simulink model "closelooprw"  (R2024a)
settings: Solver=VariableStepAuto  StartTime=0.0  StopTime=10.0  RelTol=1e-3
undefined symbols (not defined in the file or in its folder): Error_quaternio, feedback, init, motor, sat, setPoint, x
libraries: simulink x9, aerolibconvert2 x2, sharedtransform x2
settings Model: Creator=b_ant  LastModifiedBy=b_ant

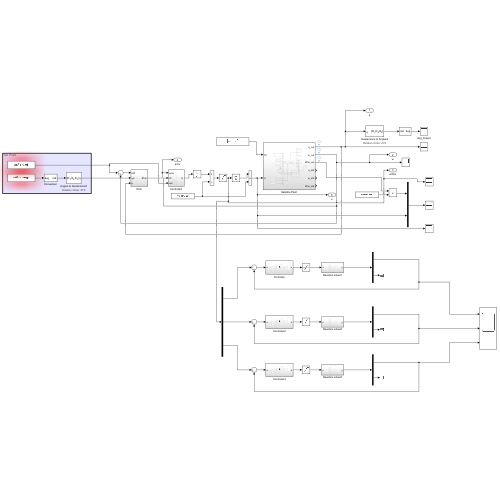
[thumbnail: Simulink's stored preview of the top-level diagram]
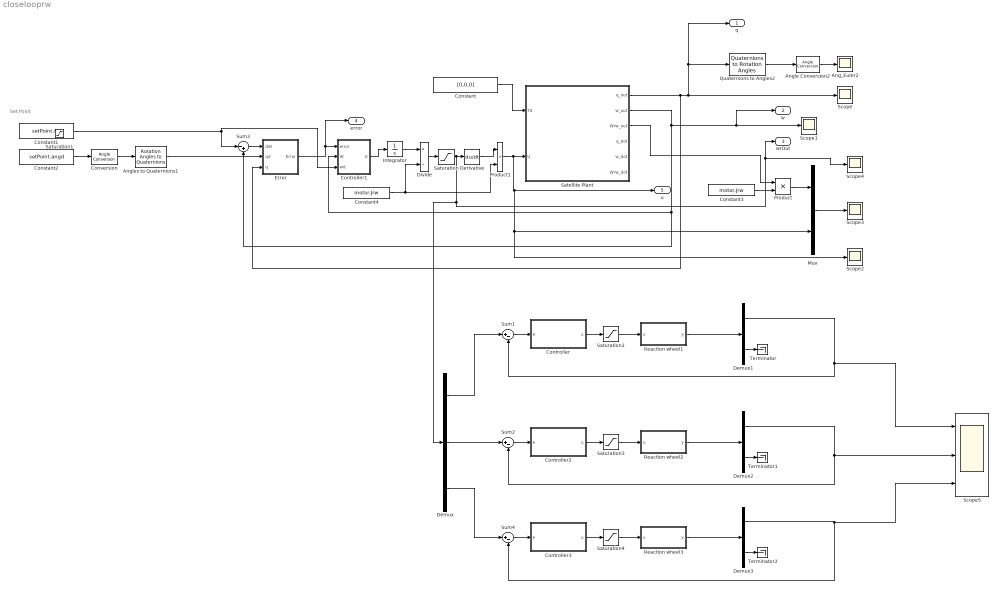
== system closelooprw ==
  note: Set Point
  Ang_Euler2 : Scope
  Angle Conversion2 : aerolibconvert2/Angle Conversion  IU=rad  OU=deg
  Angles to Quaternions1 : sharedtransform/Rotation Angles to Quaternions  rotationOrder=ZYX  aMode=aMode
  Constant : Constant  Value=[0,0,0]
  Constant1 : Constant  Value=setPoint.wd
  Constant2 : Constant  Value=setPoint.angd
  Constant3 : Constant  Value=motor.Jrw
  Constant4 : Constant  Value=motor.Jrw
  Controller : Subsystem
  Controller1 : Subsystem
  Controller2 : Subsystem
  Controller3 : Subsystem
  Conversion : aerolibconvert2/Angle Conversion  IU=deg  OU=rad
  Demux : Demux  Outputs=3
  Demux1 : Demux  Outputs=2
  Demux2 : Demux  Outputs=2
  Demux3 : Demux  Outputs=2
  Derivative : Derivative
  Divide : Product  Inputs=*/
  Error : Subsystem
  Integrator : Integrator
  Mux : Mux  Inputs=2
  Product : Product
  Product1 : Product
  Quaternions to Angles2 : sharedtransform/Quaternions to Rotation Angles  rotationOrder=ZYX  aMode=aMode
  Reaction wheel1 : Subsystem
  Reaction wheel2 : Subsystem
  Reaction wheel3 : Subsystem
  Satellite Plant : Subsystem
  Saturation : Saturate  UpperLimit=457.6253298729  LowerLimit=-457.6253298729
  Saturation{1..4} (4 alike) : Saturate  UpperLimit=12  LowerLimit=-12
  Scope{,1..4} (5 alike) : Scope
  Scope5 : Scope  NumInputPorts=3
  Sum1 : Sum  Inputs=|+-
  Sum2 : Sum  Inputs=|+-
  Sum3 : Sum  Inputs=|-+
  Sum4 : Sum  Inputs=|+-
  Terminator : Terminator
  Terminator1 : Terminator
  Terminator2 : Terminator
  q : Outport
  w : Outport  Port=2
  wrOut : Outport  Port=3
  error : Outport  Port=4
  u : Outport  Port=5
  wires:
  Reaction wheel1/1(y) -> Demux1/1
  Demux1/1 -> Scope5/1, Sum1/2
  Saturation/1 -> Demux/1, Scope4/1, wrOut/1, Derivative/1
  Sum1/1 -> Controller/1(e)
  Demux1/2 -> Terminator/1
  Derivative/1 -> Product1/1
  Product1/1 -> Scope2/1, Mux/2, u/1, Satellite Plant/2(U)
  Conversion/1 -> Angles to Quaternions1/1
  Constant/1 -> Satellite Plant/1(Td)
  Integrator/1 -> Divide/1
  Constant2/1 -> Conversion/1
  Quaternions to Angles2/1 -> Angle Conversion2/1
  Product/1 -> Mux/1
  Satellite Plant/2(w_out) -> Sum3/2, Controller1/2(W), w/1, Scope1/1
  Divide/1 -> Saturation/1
  Constant4/1 -> Product1/2, Divide/2
  Constant1/1 -> Sum3/1, Controller1/3(wd)
  Error/1(Error) -> Controller1/1(error), error/1
  Satellite Plant/3(Wrw_out) -> Product/1
  Constant3/1 -> Product/2
  Sum3/1 -> Error/1(dW)
  Controller1/1(U) -> Integrator/1
  Satellite Plant/1(q_out) -> Error/3(q), q/1, Quaternions to Angles2/1, Scope/1
  Angle Conversion2/1 -> Ang_Euler2/1
  Angles to Quaternions1/1 -> Error/2(qd)
  Mux/1 -> Scope3/1
  Controller/1(u) -> Saturation2/1
  Saturation2/1 -> Reaction wheel1/1(u)
  Controller2/1(u) -> Saturation3/1
  Saturation3/1 -> Reaction wheel2/1(u)
  Demux2/1 -> Sum2/2, Scope5/2
  Sum2/1 -> Controller2/1(e)
  Reaction wheel2/1(y) -> Demux2/1
  Controller3/1(u) -> Saturation4/1
  Saturation4/1 -> Reaction wheel3/1(u)
  Demux3/1 -> Scope5/3, Sum4/2
  Sum4/1 -> Controller3/1(e)
  Reaction wheel3/1(y) -> Demux3/1
  Demux2/2 -> Terminator1/1
  Demux3/2 -> Terminator2/1
  Demux/2 -> Sum2/1
  Demux/1 -> Sum1/1
  Demux/3 -> Sum4/1

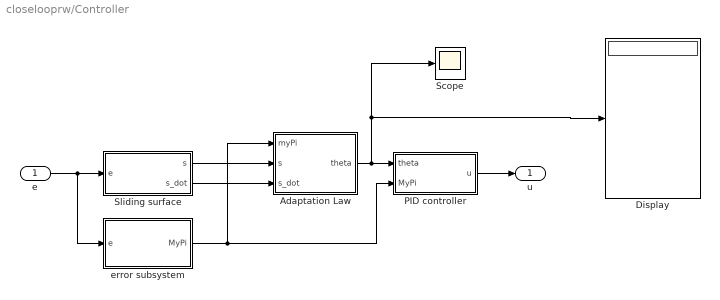
== system closelooprw/Controller ==
  e : Inport
  Adaptation Law : Subsystem  mask{alpha=x.alpha, beta=x.beta, epsilon=x.epsilon, n=x.n, kd0=x.kd_init, ki0=x.ki_init, kp0=x.kp_init}
      mask prompts: kd0 "kd_0:"; ki0 "ki_0:"; kp0 "kp_0:"
      mask TypeOptions alpha: alpha/Value
      mask TypeOptions beta: beta/Value
      mask TypeOptions epsilon: epsilon/Value
      mask TypeOptions n: n/Value
      mask TypeOptions kd0: kd0/Value
      mask TypeOptions ki0: ki0/Value
      mask TypeOptions kp0: kp0/Value
  Display : Display
  PID controller : Subsystem
  Scope : Scope
  Sliding surface : Subsystem  mask{Gain=x.lambda}
      mask prompts: Gain "Simulink:blkprm_prompts:GainGain"
      mask TypeOptions Gain: Gain/Gain
      mask DialogControl Gain Prompt: Gain:
  error subsystem : Subsystem
  u : Outport
  wires:
  Sliding surface/1(s) -> Adaptation Law/2(s)
  Sliding surface/2(s_dot) -> Adaptation Law/3(s_dot)
  PID controller/1(u) -> u/1
  Adaptation Law/1(theta) -> Scope/1, Display/1, PID controller/1(theta)
  error subsystem/1(MyPi) -> PID controller/2(MyPi), Adaptation Law/1(myPi)
  e/1 -> error subsystem/1(e), Sliding surface/1(e)

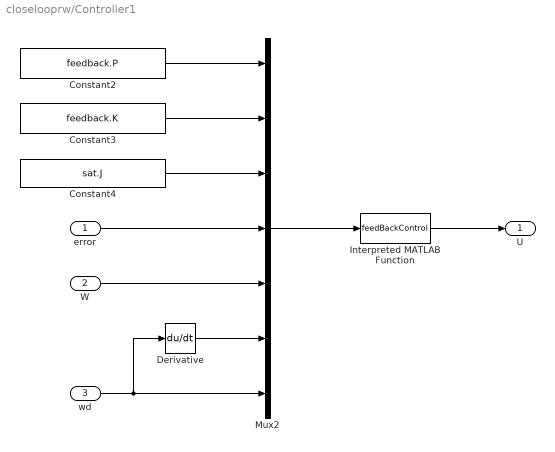
== system closelooprw/Controller1 ==
  error : Inport
  W : Inport  Port=2
  wd : Inport  Port=3
  Constant2 : Constant  Value=feedback.P
  Constant3 : Constant  Value=feedback.K
  Constant4 : Constant  Value=sat.J
  Derivative : Derivative
  Interpreted MATLAB Function : MATLABFcn  MATLABFcn=feedBackControl  OutputDimensions=3
  Mux2 : Mux  Inputs=7
  U : Outport
  wires:
  Interpreted MATLAB Function/1 -> U/1
  Constant2/1 -> Mux2/1
  Mux2/1 -> Interpreted MATLAB Function/1
  W/1 -> Mux2/5
  Constant3/1 -> Mux2/2
  error/1 -> Mux2/4
  Constant4/1 -> Mux2/3
  Derivative/1 -> Mux2/6
  wd/1 -> Derivative/1, Mux2/7

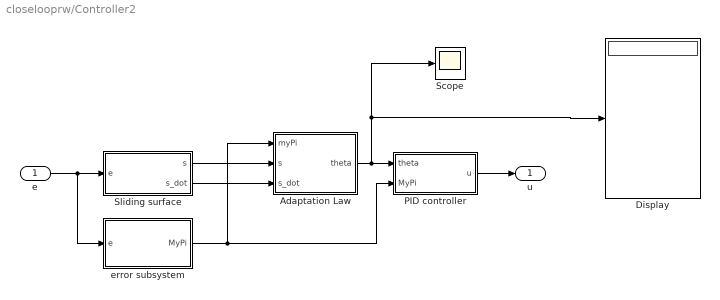
== system closelooprw/Controller2 ==
  e : Inport
  Adaptation Law : Subsystem  mask{alpha=x.alpha, beta=x.beta, epsilon=x.epsilon, n=x.n, kd0=x.kd_init, ki0=x.ki_init, kp0=x.kp_init}
      mask prompts: kd0 "kd_0:"; ki0 "ki_0:"; kp0 "kp_0:"
      mask TypeOptions alpha: alpha/Value
      mask TypeOptions beta: beta/Value
      mask TypeOptions epsilon: epsilon/Value
      mask TypeOptions n: n/Value
      mask TypeOptions kd0: kd0/Value
      mask TypeOptions ki0: ki0/Value
      mask TypeOptions kp0: kp0/Value
  Display : Display
  PID controller : Subsystem
  Scope : Scope
  Sliding surface : Subsystem  mask{Gain=x.lambda}
      mask prompts: Gain "Simulink:blkprm_prompts:GainGain"
      mask TypeOptions Gain: Gain/Gain
      mask DialogControl Gain Prompt: Gain:
  error subsystem : Subsystem
  u : Outport
  wires:
  Sliding surface/1(s) -> Adaptation Law/2(s)
  Sliding surface/2(s_dot) -> Adaptation Law/3(s_dot)
  PID controller/1(u) -> u/1
  Adaptation Law/1(theta) -> Scope/1, Display/1, PID controller/1(theta)
  error subsystem/1(MyPi) -> PID controller/2(MyPi), Adaptation Law/1(myPi)
  e/1 -> error subsystem/1(e), Sliding surface/1(e)

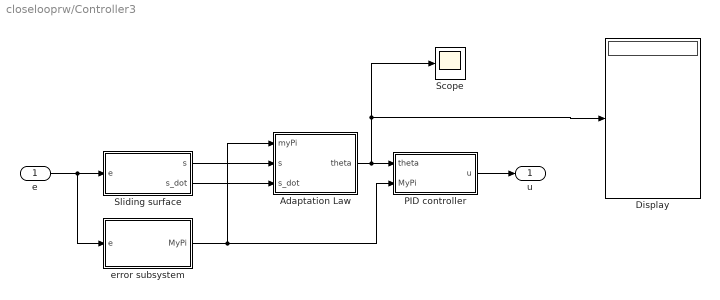
== system closelooprw/Controller3 ==
  e : Inport
  Adaptation Law : Subsystem  mask{alpha=x.alpha, beta=x.beta, epsilon=x.epsilon, n=x.n, kd0=x.kd_init, ki0=x.ki_init, kp0=x.kp_init}
      mask prompts: kd0 "kd_0:"; ki0 "ki_0:"; kp0 "kp_0:"
      mask TypeOptions alpha: alpha/Value
      mask TypeOptions beta: beta/Value
      mask TypeOptions epsilon: epsilon/Value
      mask TypeOptions n: n/Value
      mask TypeOptions kd0: kd0/Value
      mask TypeOptions ki0: ki0/Value
      mask TypeOptions kp0: kp0/Value
  Display : Display
  PID controller : Subsystem
  Scope : Scope
  Sliding surface : Subsystem  mask{Gain=x.lambda}
      mask prompts: Gain "Simulink:blkprm_prompts:GainGain"
      mask TypeOptions Gain: Gain/Gain
      mask DialogControl Gain Prompt: Gain:
  error subsystem : Subsystem
  u : Outport
  wires:
  Sliding surface/1(s) -> Adaptation Law/2(s)
  Sliding surface/2(s_dot) -> Adaptation Law/3(s_dot)
  PID controller/1(u) -> u/1
  Adaptation Law/1(theta) -> Scope/1, Display/1, PID controller/1(theta)
  error subsystem/1(MyPi) -> PID controller/2(MyPi), Adaptation Law/1(myPi)
  e/1 -> error subsystem/1(e), Sliding surface/1(e)

== system closelooprw/Error ==
  dW : Inport
  qd : Inport  Port=2
  q : Inport  Port=3
  Error quaternion : MATLABFcn  MATLABFcn=Error_quaternio(u(1),u(2),u(3),u(4),u(5),u(6),u(7),u(8))
  Mux : Mux  Inputs=2
  Mux2 : Mux  Inputs=2
  Error : Outport
  wires:
  Error quaternion/1 -> Mux/2
  Mux2/1 -> Error quaternion/1
  q/1 -> Mux2/2
  dW/1 -> Mux/1
  qd/1 -> Mux2/1
  Mux/1 -> Error/1

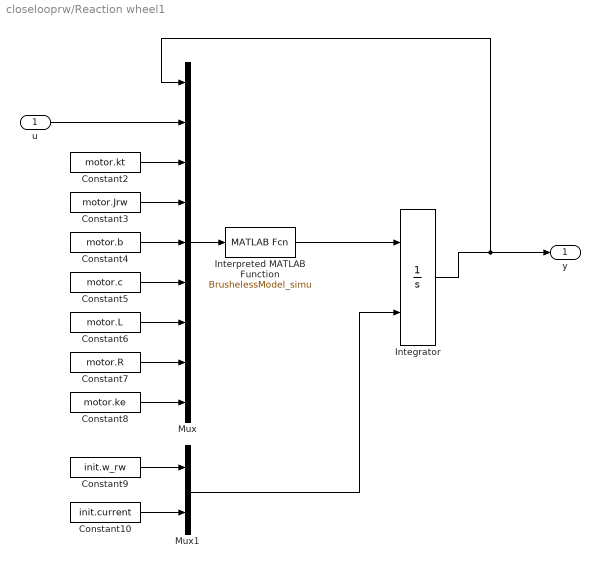
== system closelooprw/Reaction wheel1 ==
  u : Inport
  Constant10 : Constant  Value=init.current
  Constant2 : Constant  Value=motor.kt
  Constant3 : Constant  Value=motor.Jrw
  Constant4 : Constant  Value=motor.b
  Constant5 : Constant  Value=motor.c
  Constant6 : Constant  Value=motor.L
  Constant7 : Constant  Value=motor.R
  Constant8 : Constant  Value=motor.ke
  Constant9 : Constant  Value=init.w_rw
  Integrator : Integrator  InitialConditionSource=external
  Interpreted MATLAB Function : MATLABFcn  MATLABFcn=BrushelessModel_simu  OutputDimensions=2
  Mux : Mux  Inputs=9
  Mux1 : Mux  Inputs=2
  y : Outport
  wires:
  Interpreted MATLAB Function/1 -> Integrator/1
  Constant8/1 -> Mux/9
  Integrator/1 -> Mux/1, y/1
  Constant10/1 -> Mux1/2
  Constant9/1 -> Mux1/1
  Mux/1 -> Interpreted MATLAB Function/1
  Mux1/1 -> Integrator/2
  u/1 -> Mux/2
  Constant2/1 -> Mux/3
  Constant3/1 -> Mux/4
  Constant4/1 -> Mux/5
  Constant5/1 -> Mux/6
  Constant6/1 -> Mux/7
  Constant7/1 -> Mux/8

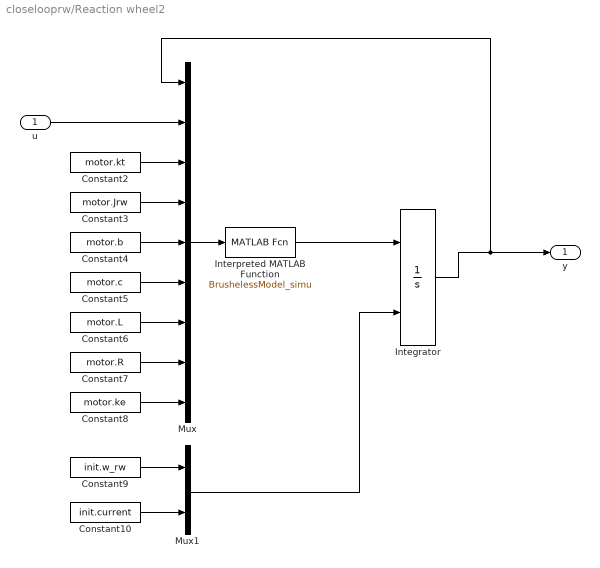
== system closelooprw/Reaction wheel2 ==
  u : Inport
  Constant10 : Constant  Value=init.current
  Constant2 : Constant  Value=motor.kt
  Constant3 : Constant  Value=motor.Jrw
  Constant4 : Constant  Value=motor.b
  Constant5 : Constant  Value=motor.c
  Constant6 : Constant  Value=motor.L
  Constant7 : Constant  Value=motor.R
  Constant8 : Constant  Value=motor.ke
  Constant9 : Constant  Value=init.w_rw
  Integrator : Integrator  InitialConditionSource=external
  Interpreted MATLAB Function : MATLABFcn  MATLABFcn=BrushelessModel_simu  OutputDimensions=2
  Mux : Mux  Inputs=9
  Mux1 : Mux  Inputs=2
  y : Outport
  wires:
  Interpreted MATLAB Function/1 -> Integrator/1
  Constant8/1 -> Mux/9
  Integrator/1 -> Mux/1, y/1
  Constant10/1 -> Mux1/2
  Constant9/1 -> Mux1/1
  Mux/1 -> Interpreted MATLAB Function/1
  Mux1/1 -> Integrator/2
  u/1 -> Mux/2
  Constant2/1 -> Mux/3
  Constant3/1 -> Mux/4
  Constant4/1 -> Mux/5
  Constant5/1 -> Mux/6
  Constant6/1 -> Mux/7
  Constant7/1 -> Mux/8

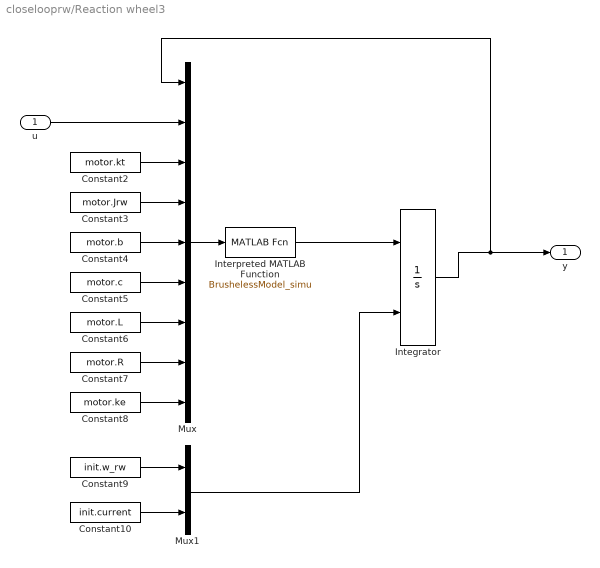
== system closelooprw/Reaction wheel3 ==
  u : Inport
  Constant10 : Constant  Value=init.current
  Constant2 : Constant  Value=motor.kt
  Constant3 : Constant  Value=motor.Jrw
  Constant4 : Constant  Value=motor.b
  Constant5 : Constant  Value=motor.c
  Constant6 : Constant  Value=motor.L
  Constant7 : Constant  Value=motor.R
  Constant8 : Constant  Value=motor.ke
  Constant9 : Constant  Value=init.w_rw
  Integrator : Integrator  InitialConditionSource=external
  Interpreted MATLAB Function : MATLABFcn  MATLABFcn=BrushelessModel_simu  OutputDimensions=2
  Mux : Mux  Inputs=9
  Mux1 : Mux  Inputs=2
  y : Outport
  wires:
  Interpreted MATLAB Function/1 -> Integrator/1
  Constant8/1 -> Mux/9
  Integrator/1 -> Mux/1, y/1
  Constant10/1 -> Mux1/2
  Constant9/1 -> Mux1/1
  Mux/1 -> Interpreted MATLAB Function/1
  Mux1/1 -> Integrator/2
  u/1 -> Mux/2
  Constant2/1 -> Mux/3
  Constant3/1 -> Mux/4
  Constant4/1 -> Mux/5
  Constant5/1 -> Mux/6
  Constant6/1 -> Mux/7
  Constant7/1 -> Mux/8

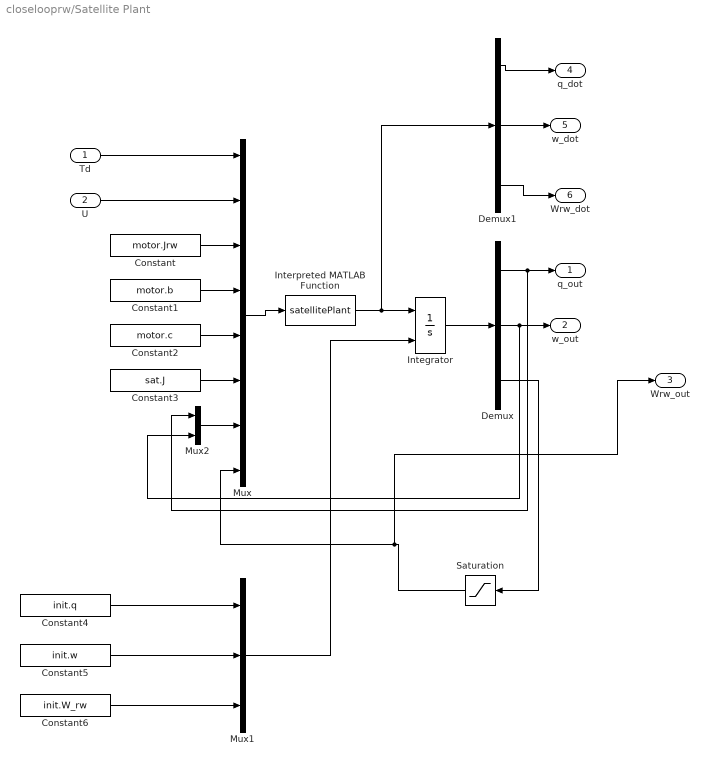
== system closelooprw/Satellite Plant ==
  Td : Inport
  U : Inport  Port=2
  Constant : Constant  Value=motor.Jrw
  Constant1 : Constant  Value=motor.b
  Constant2 : Constant  Value=motor.c
  Constant3 : Constant  Value=sat.J
  Constant4 : Constant  Value=init.q
  Constant5 : Constant  Value=init.w
  Constant6 : Constant  Value=init.W_rw
  Demux : Demux  Outputs=3
  Demux1 : Demux  Outputs=3
  Integrator : Integrator  InitialConditionSource=external
  Interpreted MATLAB Function : MATLABFcn  MATLABFcn=satellitePlant
  Mux : Mux  Inputs=8
  Mux1 : Mux  Inputs=3
  Mux2 : Mux  Inputs=2
  Saturation : Saturate  UpperLimit=457.6253298729  LowerLimit=-457.6253298729
  q_out : Outport
  w_out : Outport  Port=2
  Wrw_out : Outport  Port=3
  q_dot : Outport  Port=4
  w_dot : Outport  Port=5
  Wrw_dot : Outport  Port=6
  wires:
  Td/1 -> Mux/1
  Mux/1 -> Interpreted MATLAB Function/1
  U/1 -> Mux/2
  Interpreted MATLAB Function/1 -> Demux1/1, Integrator/1
  Constant/1 -> Mux/3
  Constant5/1 -> Mux1/2
  Constant6/1 -> Mux1/3
  Constant4/1 -> Mux1/1
  Mux1/1 -> Integrator/2
  Constant1/1 -> Mux/4
  Constant2/1 -> Mux/5
  Constant3/1 -> Mux/6
  Integrator/1 -> Demux/1
  Demux/1 -> Mux2/1, q_out/1
  Demux/2 -> Mux2/2, w_out/1
  Demux/3 -> Saturation/1
  Demux1/3 -> Wrw_dot/1
  Demux1/1 -> q_dot/1
  Demux1/2 -> w_dot/1
  Mux2/1 -> Mux/7
  Saturation/1 -> Wrw_out/1, Mux/8

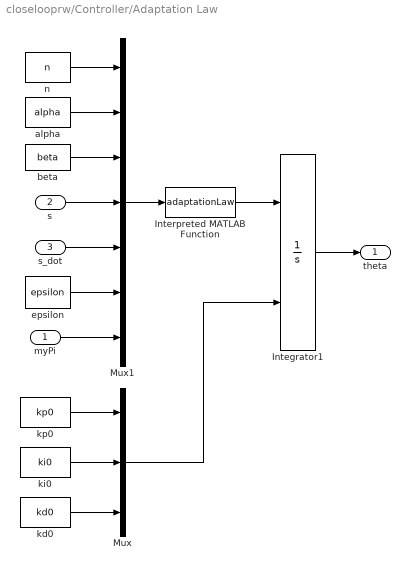
== system closelooprw/Controller/Adaptation Law ==
  myPi : Inport
  s : Inport  Port=2
  s_dot : Inport  Port=3
  Integrator1 : Integrator  InitialConditionSource=external  InitialCondition=[1.460477259865257e-04,6.548069875818259e-05,0]
  Interpreted MATLAB Function : MATLABFcn  MATLABFcn=adaptationLaw
  Mux : Mux  Inputs=3
  Mux1 : Mux  Inputs=7
  alpha : Constant  Value=alpha
  beta : Constant  Value=beta
  epsilon : Constant  Value=epsilon
  kd0 : Constant  Value=kd0
  ki0 : Constant  Value=ki0
  kp0 : Constant  Value=kp0
  n : Constant  Value=n
  theta : Outport
  wires:
  alpha/1 -> Mux1/2
  Interpreted MATLAB Function/1 -> Integrator1/1
  myPi/1 -> Mux1/7
  s/1 -> Mux1/4
  epsilon/1 -> Mux1/6
  Integrator1/1 -> theta/1
  s_dot/1 -> Mux1/5
  beta/1 -> Mux1/3
  Mux1/1 -> Interpreted MATLAB Function/1
  n/1 -> Mux1/1
  ki0/1 -> Mux/2
  Mux/1 -> Integrator1/2
  kp0/1 -> Mux/1
  kd0/1 -> Mux/3

== system closelooprw/Controller/PID controller ==
  theta : Inport
  MyPi : Inport  Port=2
  Interpreted MATLAB Function1 : MATLABFcn  MATLABFcn=controlLaw  OutputDimensions=1
  Mux2 : Mux  Inputs=2
  u : Outport
  wires:
  Mux2/1 -> Interpreted MATLAB Function1/1
  theta/1 -> Mux2/1
  Interpreted MATLAB Function1/1 -> u/1
  MyPi/1 -> Mux2/2

== system closelooprw/Controller/Sliding surface ==
  note: s
  note: e
  e : Inport
  Add : Sum
  Discrete Derivative : simulink/Discrete/Discrete Derivative  gainval=1.0  ICPrevScaledInput=0.0  OutMin=[]  OutMax=[]  OutDataType=fixdt(1, 16)  OutScaling=2^-10  DoSatur=off
  Discrete Derivative1 : simulink/Discrete/Discrete Derivative  gainval=1.0  ICPrevScaledInput=0.0  OutMin=[]  OutMax=[]  OutDataType=fixdt(1, 16)  OutScaling=2^-10  DoSatur=off
  Gain : Gain  Gain=Gain
  s : Outport
  s_dot : Outport  Port=2
  wires:
  Add/1 -> Discrete Derivative1/1, s/1
  Gain/1 -> Add/1
  e/1 -> Gain/1, Discrete Derivative/1
  Discrete Derivative/1 -> Add/2
  Discrete Derivative1/1 -> s_dot/1

== system closelooprw/Controller/error subsystem ==
  e : Inport
  Discrete Derivative : simulink/Discrete/Discrete Derivative  gainval=1.0  ICPrevScaledInput=0.0  OutMin=[]  OutMax=[]  OutDataType=fixdt(1, 16)  OutScaling=2^-10  DoSatur=off
  Integrator : Integrator
  Mux : Mux  Inputs=3
  MyPi : Outport
  wires:
  e/1 -> Mux/1, Discrete Derivative/1, Integrator/1
  Integrator/1 -> Mux/2
  Mux/1 -> MyPi/1
  Discrete Derivative/1 -> Mux/3

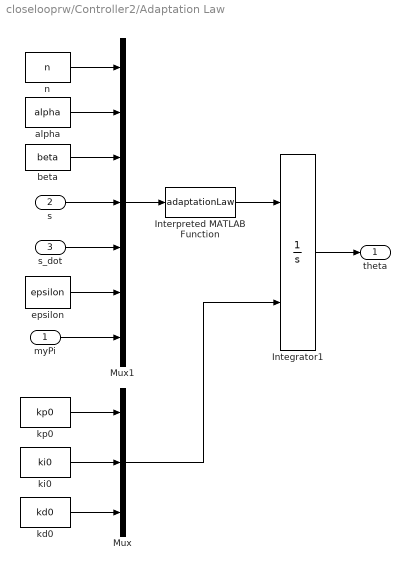
== system closelooprw/Controller2/Adaptation Law ==
  myPi : Inport
  s : Inport  Port=2
  s_dot : Inport  Port=3
  Integrator1 : Integrator  InitialConditionSource=external  InitialCondition=[1.460477259865257e-04,6.548069875818259e-05,0]
  Interpreted MATLAB Function : MATLABFcn  MATLABFcn=adaptationLaw
  Mux : Mux  Inputs=3
  Mux1 : Mux  Inputs=7
  alpha : Constant  Value=alpha
  beta : Constant  Value=beta
  epsilon : Constant  Value=epsilon
  kd0 : Constant  Value=kd0
  ki0 : Constant  Value=ki0
  kp0 : Constant  Value=kp0
  n : Constant  Value=n
  theta : Outport
  wires:
  alpha/1 -> Mux1/2
  Interpreted MATLAB Function/1 -> Integrator1/1
  myPi/1 -> Mux1/7
  s/1 -> Mux1/4
  epsilon/1 -> Mux1/6
  Integrator1/1 -> theta/1
  s_dot/1 -> Mux1/5
  beta/1 -> Mux1/3
  Mux1/1 -> Interpreted MATLAB Function/1
  n/1 -> Mux1/1
  ki0/1 -> Mux/2
  Mux/1 -> Integrator1/2
  kp0/1 -> Mux/1
  kd0/1 -> Mux/3

== system closelooprw/Controller2/PID controller ==
  theta : Inport
  MyPi : Inport  Port=2
  Interpreted MATLAB Function1 : MATLABFcn  MATLABFcn=controlLaw  OutputDimensions=1
  Mux2 : Mux  Inputs=2
  u : Outport
  wires:
  Mux2/1 -> Interpreted MATLAB Function1/1
  theta/1 -> Mux2/1
  Interpreted MATLAB Function1/1 -> u/1
  MyPi/1 -> Mux2/2

== system closelooprw/Controller2/Sliding surface ==
  note: s
  note: e
  e : Inport
  Add : Sum
  Discrete Derivative : simulink/Discrete/Discrete Derivative  gainval=1.0  ICPrevScaledInput=0.0  OutMin=[]  OutMax=[]  OutDataType=fixdt(1, 16)  OutScaling=2^-10  DoSatur=off
  Discrete Derivative1 : simulink/Discrete/Discrete Derivative  gainval=1.0  ICPrevScaledInput=0.0  OutMin=[]  OutMax=[]  OutDataType=fixdt(1, 16)  OutScaling=2^-10  DoSatur=off
  Gain : Gain  Gain=Gain
  s : Outport
  s_dot : Outport  Port=2
  wires:
  Add/1 -> Discrete Derivative1/1, s/1
  Gain/1 -> Add/1
  e/1 -> Gain/1, Discrete Derivative/1
  Discrete Derivative/1 -> Add/2
  Discrete Derivative1/1 -> s_dot/1

== system closelooprw/Controller2/error subsystem ==
  e : Inport
  Discrete Derivative : simulink/Discrete/Discrete Derivative  gainval=1.0  ICPrevScaledInput=0.0  OutMin=[]  OutMax=[]  OutDataType=fixdt(1, 16)  OutScaling=2^-10  DoSatur=off
  Integrator : Integrator
  Mux : Mux  Inputs=3
  MyPi : Outport
  wires:
  e/1 -> Mux/1, Discrete Derivative/1, Integrator/1
  Integrator/1 -> Mux/2
  Mux/1 -> MyPi/1
  Discrete Derivative/1 -> Mux/3

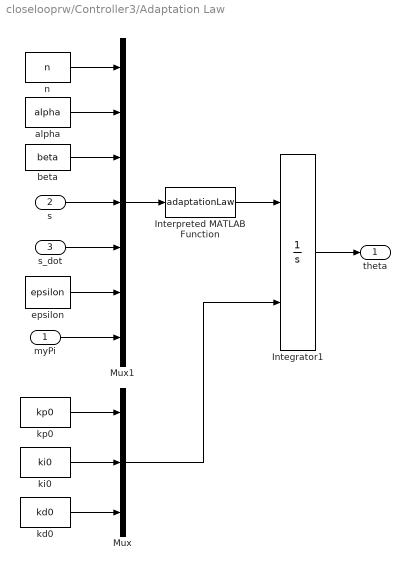
== system closelooprw/Controller3/Adaptation Law ==
  myPi : Inport
  s : Inport  Port=2
  s_dot : Inport  Port=3
  Integrator1 : Integrator  InitialConditionSource=external  InitialCondition=[1.460477259865257e-04,6.548069875818259e-05,0]
  Interpreted MATLAB Function : MATLABFcn  MATLABFcn=adaptationLaw
  Mux : Mux  Inputs=3
  Mux1 : Mux  Inputs=7
  alpha : Constant  Value=alpha
  beta : Constant  Value=beta
  epsilon : Constant  Value=epsilon
  kd0 : Constant  Value=kd0
  ki0 : Constant  Value=ki0
  kp0 : Constant  Value=kp0
  n : Constant  Value=n
  theta : Outport
  wires:
  alpha/1 -> Mux1/2
  Interpreted MATLAB Function/1 -> Integrator1/1
  myPi/1 -> Mux1/7
  s/1 -> Mux1/4
  epsilon/1 -> Mux1/6
  Integrator1/1 -> theta/1
  s_dot/1 -> Mux1/5
  beta/1 -> Mux1/3
  Mux1/1 -> Interpreted MATLAB Function/1
  n/1 -> Mux1/1
  ki0/1 -> Mux/2
  Mux/1 -> Integrator1/2
  kp0/1 -> Mux/1
  kd0/1 -> Mux/3

== system closelooprw/Controller3/PID controller ==
  theta : Inport
  MyPi : Inport  Port=2
  Interpreted MATLAB Function1 : MATLABFcn  MATLABFcn=controlLaw  OutputDimensions=1
  Mux2 : Mux  Inputs=2
  u : Outport
  wires:
  Mux2/1 -> Interpreted MATLAB Function1/1
  theta/1 -> Mux2/1
  Interpreted MATLAB Function1/1 -> u/1
  MyPi/1 -> Mux2/2

== system closelooprw/Controller3/Sliding surface ==
  note: s
  note: e
  e : Inport
  Add : Sum
  Discrete Derivative : simulink/Discrete/Discrete Derivative  gainval=1.0  ICPrevScaledInput=0.0  OutMin=[]  OutMax=[]  OutDataType=fixdt(1, 16)  OutScaling=2^-10  DoSatur=off
  Discrete Derivative1 : simulink/Discrete/Discrete Derivative  gainval=1.0  ICPrevScaledInput=0.0  OutMin=[]  OutMax=[]  OutDataType=fixdt(1, 16)  OutScaling=2^-10  DoSatur=off
  Gain : Gain  Gain=Gain
  s : Outport
  s_dot : Outport  Port=2
  wires:
  Add/1 -> Discrete Derivative1/1, s/1
  Gain/1 -> Add/1
  e/1 -> Gain/1, Discrete Derivative/1
  Discrete Derivative/1 -> Add/2
  Discrete Derivative1/1 -> s_dot/1

== system closelooprw/Controller3/error subsystem ==
  e : Inport
  Discrete Derivative : simulink/Discrete/Discrete Derivative  gainval=1.0  ICPrevScaledInput=0.0  OutMin=[]  OutMax=[]  OutDataType=fixdt(1, 16)  OutScaling=2^-10  DoSatur=off
  Integrator : Integrator
  Mux : Mux  Inputs=3
  MyPi : Outport
  wires:
  e/1 -> Mux/1, Discrete Derivative/1, Integrator/1
  Integrator/1 -> Mux/2
  Mux/1 -> MyPi/1
  Discrete Derivative/1 -> Mux/3
